simulink model "Final"  (R2018a)
settings: Solver=ode4  StartTime=0.0  StopTime=inf  FixedStep=0.01  RelTol=1e-3  EnableMultiTasking=on
model workspace (MAT data in the model file):
  Kp = 1
settings Model: ExtModeTrigDuration=5000  ParameterArgumentNames=Kp  OrderedModelArguments=off  Creator=benmiao  LastModifiedBy=benmiao
settings SolverCC: PositivePriorityOrder=on
settings DataIOCC: LimitDataPoints=on  SaveFormat=Array
settings OptimizationCC: ExpressionDepthLimit=2147483647  LifeSpan=inf
settings DebuggingCC: UnderspecifiedInitializationDetection=Classic  MergeDetectMultiDrivingBlocksExec=none  SolverPrmCheckMsg=warning  StateNameClashWarn=warning  SFUnexpectedBacktrackingDiag=warning  SFNoUnconditionalDefaultTransitionDiag=warning  SFExecutionAtInitializationDiag=none
settings HardwareCC: ProdBitPerPointer=32  ProdBitPerSizeT=32  ProdBitPerPtrDiffT=32  ProdLargestAtomicFloat=None  ProdIntDivRoundTo=Undefined  ProdEndianess=Unspecified  ProdWordSize=32  ProdHWDeviceType=32-bit Generic
settings ModelReferenceCC: PropagateSignalLabelsOutOfModel=off
settings RTWCC: SystemTargetFile=quarc_win64.tlc  TemplateMakefile=quarc_default_tmf  Description=QUARC Win64 Target
settings CodeAppCC: StateflowObjectComments=on
settings STFCustomTargetCC: TargetPreCompLibLocation=C:\PROGRA~3\QUARC\lib\2012b\win64\release  GeneratePreprocessorConditionals=Disable all  CombineOutputUpdateFcns=on  CPPClassGenCompliant=on  GRTInterface=off  SystemTargetFile=quarc_win64.tlc
settings GRTTargetCC: TargetPreCompLibLocation=C:\PROGRA~3\QUARC\lib\2012b\win64\release  TargetLangStandard=C89/C90 (ANSI)  ParMdlRefBuildCompliant=off  CompOptLevelCompliant=off  ConcurrentExecutionCompliant=off  GeneratePreprocessorConditionals=Disable all  MatFileLogging=off  UseToolchainInfoCompliant=off  ExtMode=on  ExtModeMexFile=quarc_comm
settings ConfigComp: CovMetricSettings=dw  CovHtmlReporting=on  CovSaveCumulativeToWorkspaceVar=on  CovSaveSingleToWorkspaceVar=on  CovExternalEMLEnable=off

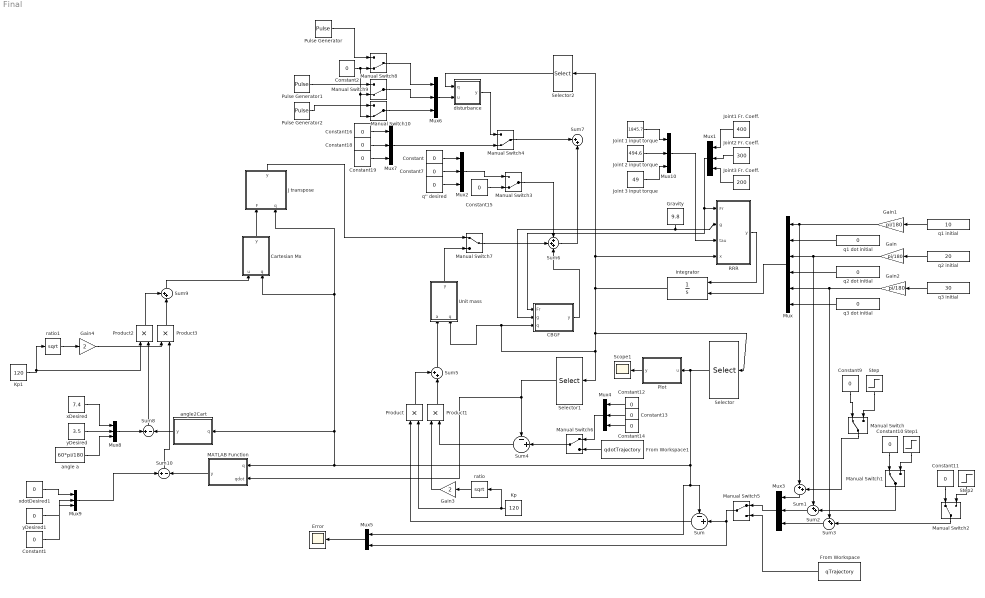
== system Final ==
  CBGF : MATLAB Function  TreatAsAtomicUnit=on
  Cartesian Mx : MATLAB Function  TreatAsAtomicUnit=on
  Constant{,1..2,7,9..16,18..19} (14 alike) : Constant  Value=0
  Error : Scope
  From Workspace : FromWorkspace  VariableName=qTrajectory  SampleTime=0
  From Workspace1 : FromWorkspace  VariableName=qdotTrajectory  SampleTime=0
  Gain : Gain  Gain=pi/180
  Gain1 : Gain  Gain=pi/180
  Gain2 : Gain  Gain=pi/180
  Gain3 : Gain  Gain=2
  Gain4 : Gain  Gain=2
  Gravity : Constant  Value=9.8
  Integrator : Integrator  InitialConditionSource=external
  J transpose : MATLAB Function  TreatAsAtomicUnit=on
  Joint 1 input torque : Constant  Value=1845.7
  Joint 2 input torque : Constant  Value=494.6
  Joint 3 input torque : Constant  Value=49
  Joint1 Fr. Coeff. : Constant  Value=400
  Joint2 Fr. Coeff. : Constant  Value=300
  Joint3 Fr. Coeff. : Constant  Value=200
  Kp : Constant  Value=120
  Kp1 : Constant  Value=120
  MATLAB Function : MATLAB Function  TreatAsAtomicUnit=on
  Manual Switch{,1..2,5..7} (6 alike) : ManualSwitch
  Manual Switch{3..4,8..10} (5 alike) : ManualSwitch  CurrentSetting=0
  Mux : Mux  Inputs=6
  Mux{1..4,6..10} (9 alike) : Mux  Inputs=3
  Mux5 : Mux  Inputs=2
  Plot : MATLAB Function  TreatAsAtomicUnit=on
  Product{,1..3} (4 alike) : Product
  Pulse Generator : DiscretePulseGenerator  PulseType=Time based  Amplitude=200  Period=5  PulseWidth=5
  Pulse Generator1 : DiscretePulseGenerator  PulseType=Time based  Amplitude=200  Period=5  PulseWidth=5
  Pulse Generator2 : DiscretePulseGenerator  PulseType=Time based  Amplitude=200  Period=5  PulseWidth=5
  RRR : MATLAB Function  TreatAsAtomicUnit=on
  Scope1 : Scope
  Selector : Selector  InputPortWidth=6  IndexOptions=Index vector (dialog)  Indices=[1 3 5]  OutputSizes=1
  Selector1 : Selector  InputPortWidth=6  IndexOptions=Index vector (dialog)  Indices=[2 4 6]  OutputSizes=1
  Selector2 : Selector  InputPortWidth=6  IndexOptions=Index vector (dialog)  Indices=[1 3 5]  OutputSizes=1
  Step : Step  Time=0  After=pi/18  SampleTime=0
  Step1 : Step  Time=0  After=pi/18  SampleTime=0
  Step2 : Step  Time=0  After=pi/2  SampleTime=0
  Sum : Sum  Inputs=-+|
  Sum1 : Sum  Inputs=|++
  Sum10 : Sum  Inputs=+|-
  Sum{2..3,5,9} (4 alike) : Sum  Inputs=++|
  Sum4 : Sum  Inputs=-+|
  Sum6 : Sum  Inputs=+++
  Sum7 : Sum  Inputs=|++
  Sum8 : Sum  Inputs=+|-
  Unit mass : MATLAB Function  TreatAsAtomicUnit=on
  angle a : Constant  Value=60*pi/180
  angle2Cart : MATLAB Function  TreatAsAtomicUnit=on
  disturbance : MATLAB Function  TreatAsAtomicUnit=on
  q'' desired : Constant  Value=0
  q1 dot initial : Constant  Value=0
  q1 initial : Constant  Value=10
  q2 dot initial : Constant  Value=0
  q2 initial : Constant  Value=20
  q3 dot initial : Constant  Value=0
  q3 initial : Constant  Value=30
  ratio : Sqrt  SaturateOnIntegerOverflow=on
  ratio1 : Sqrt  SaturateOnIntegerOverflow=on
  xDesired : Constant  Value=7.4
  xdotDesired1 : Constant  Value=0
  yDesired : Constant  Value=3.5
  yDesired1 : Constant  Value=0
  wires:
  q1 initial/1 -> Gain1/1
  q1 dot initial/1 -> Mux/2
  q2 dot initial/1 -> Mux/4
  q3 initial/1 -> Gain2/1
  q3 dot initial/1 -> Mux/6
  RRR/1(y) -> Integrator/1
  Gravity/1 -> CBGF/2(g), RRR/2(g)
  Selector/1 -> Sum/1, Mux5/1, Cartesian Mx/2(q), J transpose/2(q), angle2Cart/1(q), MATLAB Function/1(q), Plot/1(u)
  Integrator/1 -> Selector2/1, RRR/4(x), CBGF/3(q), Unit mass/2(q), Selector1/1, Selector/1
  Mux1/1 -> CBGF/1(Fr), RRR/1(Fr)
  Plot/1(y) -> Scope1/1
  Constant/1 -> Mux2/1
  Constant7/1 -> Mux2/2
  q'' desired/1 -> Mux2/3
  Mux/1 -> Integrator/2
  Joint1 Fr. Coeff./1 -> Mux1/1
  Joint2 Fr. Coeff./1 -> Mux1/2
  Joint3 Fr. Coeff./1 -> Mux1/3
  Sum/1 -> Product/1
  Step/1 -> Manual Switch/2
  Manual Switch/1 -> Sum1/2
  Constant9/1 -> Manual Switch/1
  Sum1/1 -> Mux3/1
  Constant10/1 -> Manual Switch1/1
  Step1/1 -> Manual Switch1/2
  Manual Switch1/1 -> Sum2/2
  Sum2/1 -> Mux3/2
  Constant11/1 -> Manual Switch2/1
  Step2/1 -> Manual Switch2/2
  Manual Switch2/1 -> Sum3/2
  Sum3/1 -> Mux3/3
  Constant12/1 -> Mux4/1
  Constant13/1 -> Mux4/2
  Constant14/1 -> Mux4/3
  Mux4/1 -> Manual Switch6/1
  Selector1/1 -> MATLAB Function/2(qdot), Sum4/1
  Gain1/1 -> Sum1/1, Mux/1
  q2 initial/1 -> Gain/1
  Gain/1 -> Mux/3, Sum2/1
  Gain2/1 -> Mux/5, Sum3/1
  Sum5/1 -> Unit mass/1(a)
  Unit mass/1(y) -> Manual Switch7/2
  CBGF/1(y) -> Sum6/3
  Mux2/1 -> Manual Switch3/1
  Sum4/1 -> Product1/2
  Kp/1 -> ratio/1, Product/2
  Product/1 -> Sum5/1
  Product1/1 -> Sum5/2
  Constant15/1 -> Manual Switch3/2
  Manual Switch3/1 -> Sum6/1
  Mux5/1 -> Error/1
  Gain3/1 -> Product1/1
  Sum6/1 -> Sum7/2
  Mux6/1 -> disturbance/2(u)
  Mux10/1 -> RRR/3(tau)
  ratio/1 -> Gain3/1
  Mux3/1 -> Manual Switch5/1
  Manual Switch5/1 -> Mux5/2, Sum/2
  From Workspace/1 -> Manual Switch5/2
  From Workspace1/1 -> Manual Switch6/2
  Manual Switch6/1 -> Sum4/2
  Selector2/1 -> disturbance/1(q)
  Mux7/1 -> Manual Switch4/2
  Constant18/1 -> Mux7/2
  Constant19/1 -> Mux7/3
  Constant16/1 -> Mux7/1
  disturbance/1(y) -> Manual Switch4/1
  Manual Switch4/1 -> Sum7/1
  Pulse Generator/1 -> Manual Switch8/1
  xDesired/1 -> Mux8/1
  yDesired/1 -> Mux8/2
  angle a/1 -> Mux8/3
  Mux8/1 -> Sum8/1
  angle2Cart/1(y) -> Sum8/2
  Cartesian Mx/1(y) -> J transpose/1(F)
  J transpose/1(y) -> Manual Switch7/1
  Manual Switch7/1 -> Sum6/2
  ratio1/1 -> Gain4/1
  Product3/1 -> Sum9/2
  Product2/1 -> Sum9/1
  Sum9/1 -> Cartesian Mx/1(u)
  Gain4/1 -> Product3/1
  MATLAB Function/1(y) -> Sum10/2
  xdotDesired1/1 -> Mux9/1
  Constant1/1 -> Mux9/3
  yDesired1/1 -> Mux9/2
  Mux9/1 -> Sum10/1
  Sum8/1 -> Product2/2
  Sum10/1 -> Product3/2
  Kp1/1 -> ratio1/1, Product2/1
  Pulse Generator1/1 -> Manual Switch9/1
  Pulse Generator2/1 -> Manual Switch10/1
  Manual Switch8/1 -> Mux6/1
  Manual Switch9/1 -> Mux6/2
  Manual Switch10/1 -> Mux6/3
  Constant2/1 -> Manual Switch9/2, Manual Switch10/2, Manual Switch8/2
  Joint 2 input torque/1 -> Mux10/2
  Joint 3 input torque/1 -> Mux10/3
  Joint 1 input torque/1 -> Mux10/1

== matlab function Final/Plot ==
  data: y output; u input
function y = fcn(u)
%
% q1 = u(1);
% q2 = u(2);
% q3 = u(3);
%
% x0 = 0;
% y0 = 0;
% x1 = 4*cos( q1);
% y1 = 4*sin( q1);
%
% x2 = 3*cos( (q1+q2));
% y2 = 3*sin( (q1+q2));
%
% x3 = 2*cos( (q1+q2+q3));
% y3 = 2*sin( (q1+q2+q3));
%
% px0= 0;
% py0 = 0;
% px1 = x1;
% py1 = y1;
% px2 = x1+x2;
% py2 = y1+y2;
% px3 = x1+x2+x3;
% py3 = y1+y2+y3;
%
% plot([px0,px1,px2,px3],[py0,py1,py2,py3]);
% xlim([-10,10]);
% ylim([-10,10]);
%
y = u;
q1 = u(1);
q2 = u(2);
q3 = u(3);
L1 = 4;
L2 = 3;
L3 = 2;

link11_end = [4;0;0;1];
link11_start = [0;0;0;1];
link22_end = [3;0;0;1];
link33_end = [2;0;0;1];
linkE3_end1 = [2;0.5;0;1];
linkE3_end2 = [2.5;0.5;0;1];
linkE3_end3 = [2;-0.5;0;1];
linkE3_end4 = [2.5;-0.5;0;1];


T_01 = [cos(q1) -sin(q1) 0 0;
    sin(q1) cos(q1) 0 0;
    0 0 1 0;
    0 0 0 1];

T_02 = [cos(q1+q2) -sin(q1+q2) 0 L1*cos(q1);
    sin(q1+q2) cos(q1+q2) 0 L1*sin(q1);
    0 0 1 0;
    0 0 0 1];

T_03 = [cos(q1+q2+q3) -sin(q1+q2+q3) 0 L2*cos(q1+q2)+L1*cos(q1);
    sin(q1+q2+q3) cos(q1+q2+q3) 0 L2*sin(q1+q2)+L1*sin(q1);
    0 0 1 0;
    0 0 0 1];

link10_end = T_01* link11_end;
link10_start = T_01* link11_start;

link20_end = T_02 * link22_end;

link30_end = T_03 * link33_end;

linkE0_end1 = T_03 * linkE3_end1;
linkE0_end2 = T_03 * linkE3_end2;
linkE0_end3 = T_03 * linkE3_end3;
linkE0_end4 = T_03 * linkE3_end4;

% plot([link10_start(1),link10_end(1),link20_end(1),link30_end(1),linkE0_end1(1),linkE0_end2(1),linkE0_end1(1),linkE0_end3(1),linkE0_end4(1)], ...
% [link10_start(2),link10_end(2),link20_end(2),link30_end(2),linkE0_end1(2),linkE0_end2(2),linkE0_end1(2),linkE0_end3(2),linkE0_end4(2)]);

plot([link10_start(1),link10_end(1)],[link10_start(2),link10_end(2)],'k');

hold on;
plot([link10_end(1),link20_end(1)],[link10_end(2),link20_end(2)],'m');

plot([link20_end(1),link30_end(1)],[link20_end(2),link30_end(2)],'b');

plot([link30_end(1),linkE0_end1(1),linkE0_end2(1),linkE0_end1(1),linkE0_end3(1),linkE0_end4(1)], ...
    [link30_end(2),linkE0_end1(2),linkE0_end2(2),linkE0_end1(2),linkE0_end3(2),linkE0_end4(2)],'c');

hold off;
grid on
xlim([-10,10]);
ylim([-10,10]);
title('RRR Robot Simulation');
xlabel('x Position');
ylabel('y Position');
end

== matlab function Final/RRR ==
  data: Fr input; g input; tau input; x input; y output

function y = fcn(Fr,g,tau,x)

q1 = x(1);
q2 = x(3);
q3 = x(5);

M = zeros(3);
M = [80*cos(q2 + q3) + 420*cos(q2) + 60*cos(q3) + 12291/20, 40*cos(q2 + q3) + 210*cos(q2) + 60*cos(q3) + 2681/20, 40*cos(q2 + q3) + 30*cos(q3) + 101/10;
    40*cos(q2 + q3) + 210*cos(q2) + 60*cos(q3) + 2681/20,                                 60*cos(q3) + 2681/20,                   30*cos(q3) + 101/10;
    40*cos(q2 + q3) + 30*cos(q3) + 101/10,                                  30*cos(q3) + 101/10,                                101/10];

B = zeros(3);
B = [ - 80*sin(q2 + q3) - 420*sin(q2), - 80*sin(q2 + q3) - 60*sin(q3), - 80*sin(q2 + q3) - 60*sin(q3);
    0,                    -60*sin(q3),                    -60*sin(q3);
    60*sin(q3),                              0,                              0];

C= zeros(3);
C = [                             0, - 40*sin(q2 + q3) - 210*sin(q2), - 40*sin(q2 + q3) - 30*sin(q3);
    40*sin(q2 + q3) + 210*sin(q2),                               0,                    -30*sin(q3);
    40*sin(q2 + q3) + 30*sin(q3),                      30*sin(q3),                              0];

G = [0;0;0];
G = [15*g*((3*cos(q1 + q2))/2 + 4*cos(q1)) + 10*g*(cos(q1 + q2 + q3) + 3*cos(q1 + q2) + 4*cos(q1)) + 40*g*cos(q1);
    10*g*(cos(q1 + q2 + q3) + 3*cos(q1 + q2)) + (45*g*cos(q1 + q2))/2;
    10*g*cos(q1 + q2 + q3)];

F = Fr .* [x(2);x(4);x(6)];

qdotdot = M\(tau -   C*[x(2)^2;x(4)^2;x(6)^2] - B*[ x(2)*x(4); x(2)*x(6); x(4)*x(6)] - G - F);
torque = C*[x(2)^2;x(4)^2;x(6)^2]+ B*[ x(2)*x(4); x(2)*x(6); x(4)*x(6)] + G

y = [x(2);
    qdotdot(1);
    x(4);
    qdotdot(2);
    x(6);
    qdotdot(3)];
end

== matlab function Final/Unit mass ==
  data: a input; y output; q input
function y = fcn(a,q)
q1 = q(1);
q2 = q(3);
q3 = q(5);

M = zeros(3);
M = [80*cos(q2 + q3) + 420*cos(q2) + 60*cos(q3) + 12291/20, 40*cos(q2 + q3) + 210*cos(q2) + 60*cos(q3) + 2681/20, 40*cos(q2 + q3) + 30*cos(q3) + 101/10;
    40*cos(q2 + q3) + 210*cos(q2) + 60*cos(q3) + 2681/20,                                 60*cos(q3) + 2681/20,                   30*cos(q3) + 101/10;
    40*cos(q2 + q3) + 30*cos(q3) + 101/10,                                  30*cos(q3) + 101/10,                                101/10];

y = M*a;
end

== matlab function Final/CBGF ==
  data: Fr input; y output; g input; q input
function y = fcn(Fr,g,q)
q1 = q(1);
q2 = q(3);
q3 = q(5);

M = zeros(3);
M = [80*cos(q2 + q3) + 420*cos(q2) + 60*cos(q3) + 12291/20, 40*cos(q2 + q3) + 210*cos(q2) + 60*cos(q3) + 2681/20, 40*cos(q2 + q3) + 30*cos(q3) + 101/10;
    40*cos(q2 + q3) + 210*cos(q2) + 60*cos(q3) + 2681/20,                                 60*cos(q3) + 2681/20,                   30*cos(q3) + 101/10;
    40*cos(q2 + q3) + 30*cos(q3) + 101/10,                                  30*cos(q3) + 101/10,                                101/10];

B = zeros(3);
B = [ - 80*sin(q2 + q3) - 420*sin(q2), - 80*sin(q2 + q3) - 60*sin(q3), - 80*sin(q2 + q3) - 60*sin(q3);
    0,                    -60*sin(q3),                    -60*sin(q3);
    60*sin(q3),                              0,                              0];

C= zeros(3);
C = [                             0, - 40*sin(q2 + q3) - 210*sin(q2), - 40*sin(q2 + q3) - 30*sin(q3);
    40*sin(q2 + q3) + 210*sin(q2),                               0,                    -30*sin(q3);
    40*sin(q2 + q3) + 30*sin(q3),                      30*sin(q3),                              0];

G = [0;0;0];
G = [15*g*((3*cos(q1 + q2))/2 + 4*cos(q1)) + 10*g*(cos(q1 + q2 + q3) + 3*cos(q1 + q2) + 4*cos(q1)) + 40*g*cos(q1);
    10*g*(cos(q1 + q2 + q3) + 3*cos(q1 + q2)) + (45*g*cos(q1 + q2))/2;
    10*g*cos(q1 + q2 + q3)];

F = Fr .* [q(2);q(4);q(6)];

y = C*[q(2)^2;q(4)^2;q(6)^2] + B*[ q(2)*q(4); q(2)*q(6); q(4)*q(6)] + G + F;

== matlab function Final/disturbance ==
  data: q input; u input; y output
function y = fcn(q,u)
L1 = 4;
L2 = 3;
L3 = 2;

q1 = q(1);
q2 = q(2);
q3 = q(3);

J0 = [-L3*sin(q1+q2+q3)-L2*sin(q1+q2)-L1*sin(q1) -L3*sin(q1+q2+q3)-L2*sin(q1+q2) -L3*sin(q1+q2+q3);
    L3*cos(q1+q2+q3)+L2*cos(q1+q2)+L1*cos(q1) L3*cos(q1+q2+q3)+L2*cos(q1+q2) L3*cos(q1+q2+q3);
    1 0 0];


y = J0.' * u;

== matlab function Final/Cartesian Mx ==
  data: u input; y output; q input
function y = mx(u,q)
q1 = q(1);
q2 = q(2);
q3 = q(3);
Mx = [                                                                                                                                                                                                                                                                                                                                                                                                                                                                                (((101*(2*cos(q1 + q2 + q3) + 3*cos(q1 + q2)))/(60*(cos(q1 + q2 + q3)*sin(q1 + q2) - sin(q1 + q2 + q3)*cos(q1 + q2))) - (cos(q1 + q2 + q3)*(30*cos(q3) + 101/10))/(3*(cos(q1 + q2 + q3)*sin(q1 + q2) - sin(q1 + q2 + q3)*cos(q1 + q2))))*(2*cos(q1 + q2 + q3) + 3*cos(q1 + q2)))/(6*(cos(q1 + q2 + q3)*sin(q1 + q2) - sin(q1 + q2 + q3)*cos(q1 + q2))) + (cos(q1 + q2 + q3)*((cos(q1 + q2 + q3)*(60*cos(q3) + 2681/20))/(3*(cos(q1 + q2 + q3)*sin(q1 + q2) - sin(q1 + q2 + q3)*cos(q1 + q2))) - ((30*cos(q3) + 101/10)*(2*cos(q1 + q2 + q3) + 3*cos(q1 + q2)))/(6*(cos(q1 + q2 + q3)*sin(q1 + q2) - sin(q1 + q2 + q3)*cos(q1 + q2)))))/(3*(cos(q1 + q2 + q3)*sin(q1 + q2) - sin(q1 + q2 + q3)*cos(q1 + q2))),                                                                                                                                                                                                                                                                                                                                                                                                                                                                                (((101*(2*cos(q1 + q2 + q3) + 3*cos(q1 + q2)))/(60*(cos(q1 + q2 + q3)*sin(q1 + q2) - sin(q1 + q2 + q3)*cos(q1 + q2))) - (cos(q1 + q2 + q3)*(30*cos(q3) + 101/10))/(3*(cos(q1 + q2 + q3)*sin(q1 + q2) - sin(q1 + q2 + q3)*cos(q1 + q2))))*(2*sin(q1 + q2 + q3) + 3*sin(q1 + q2)))/(6*(cos(q1 + q2 + q3)*sin(q1 + q2) - sin(q1 + q2 + q3)*cos(q1 + q2))) + (sin(q1 + q2 + q3)*((cos(q1 + q2 + q3)*(60*cos(q3) + 2681/20))/(3*(cos(q1 + q2 + q3)*sin(q1 + q2) - sin(q1 + q2 + q3)*cos(q1 + q2))) - ((30*cos(q3) + 101/10)*(2*cos(q1 + q2 + q3) + 3*cos(q1 + q2)))/(6*(cos(q1 + q2 + q3)*sin(q1 + q2) - sin(q1 + q2 + q3)*cos(q1 + q2)))))/(3*(cos(q1 + q2 + q3)*sin(q1 + q2) - sin(q1 + q2 + q3)*cos(q1 + q2))),                                                                                                                                                                                                                                                                                                                                                                                                                                                                                                                                                                                                                                                                                                                                 (2*((101*(2*cos(q1 + q2 + q3) + 3*cos(q1 + q2)))/(60*(cos(q1 + q2 + q3)*sin(q1 + q2) - sin(q1 + q2 + q3)*cos(q1 + q2))) - (cos(q1 + q2 + q3)*(30*cos(q3) + 101/10))/(3*(cos(q1 + q2 + q3)*sin(q1 + q2) - sin(q1 + q2 + q3)*cos(q1 + q2))))*(2*cos(q1 + q2 + q3)*sin(q1) - 2*sin(q1 + q2 + q3)*cos(q1) + 3*cos(q1 + q2)*sin(q1) - 3*sin(q1 + q2)*cos(q1)))/(3*(cos(q1 + q2 + q3)*sin(q1 + q2) - sin(q1 + q2 + q3)*cos(q1 + q2))) + (((cos(q1 + q2 + q3)*(60*cos(q3) + 2681/20))/(3*(cos(q1 + q2 + q3)*sin(q1 + q2) - sin(q1 + q2 + q3)*cos(q1 + q2))) - ((30*cos(q3) + 101/10)*(2*cos(q1 + q2 + q3) + 3*cos(q1 + q2)))/(6*(cos(q1 + q2 + q3)*sin(q1 + q2) - sin(q1 + q2 + q3)*cos(q1 + q2))))*(3*cos(q1 + q2 + q3)*sin(q1 + q2) - 3*sin(q1 + q2 + q3)*cos(q1 + q2) + 4*cos(q1 + q2 + q3)*sin(q1) - 4*sin(q1 + q2 + q3)*cos(q1)))/(3*(cos(q1 + q2 + q3)*sin(q1 + q2) - sin(q1 + q2 + q3)*cos(q1 + q2))) - (cos(q1 + q2 + q3)*(40*cos(q2 + q3) + 210*cos(q2) + 60*cos(q3) + 2681/20))/(3*(cos(q1 + q2 + q3)*sin(q1 + q2) - sin(q1 + q2 + q3)*cos(q1 + q2))) + ((2*cos(q1 + q2 + q3) + 3*cos(q1 + q2))*(40*cos(q2 + q3) + 30*cos(q3) + 101/10))/(6*(cos(q1 + q2 + q3)*sin(q1 + q2) - sin(q1 + q2 + q3)*cos(q1 + q2)));
                                                                                                                                                                                                                                                                                                                                                                                                                                                                                (cos(q1 + q2 + q3)*((sin(q1 + q2 + q3)*(60*cos(q3) + 2681/20))/(3*(cos(q1 + q2 + q3)*sin(q1 + q2) - sin(q1 + q2 + q3)*cos(q1 + q2))) - ((30*cos(q3) + 101/10)*(2*sin(q1 + q2 + q3) + 3*sin(q1 + q2)))/(6*(cos(q1 + q2 + q3)*sin(q1 + q2) - sin(q1 + q2 + q3)*cos(q1 + q2)))))/(3*(cos(q1 + q2 + q3)*sin(q1 + q2) - sin(q1 + q2 + q3)*cos(q1 + q2))) + ((2*cos(q1 + q2 + q3) + 3*cos(q1 + q2))*((101*(2*sin(q1 + q2 + q3) + 3*sin(q1 + q2)))/(60*(cos(q1 + q2 + q3)*sin(q1 + q2) - sin(q1 + q2 + q3)*cos(q1 + q2))) - (sin(q1 + q2 + q3)*(30*cos(q3) + 101/10))/(3*(cos(q1 + q2 + q3)*sin(q1 + q2) - sin(q1 + q2 + q3)*cos(q1 + q2)))))/(6*(cos(q1 + q2 + q3)*sin(q1 + q2) - sin(q1 + q2 + q3)*cos(q1 + q2))),                                                                                                                                                                                                                                                                                                                                                                                                                                                                                (sin(q1 + q2 + q3)*((sin(q1 + q2 + q3)*(60*cos(q3) + 2681/20))/(3*(cos(q1 + q2 + q3)*sin(q1 + q2) - sin(q1 + q2 + q3)*cos(q1 + q2))) - ((30*cos(q3) + 101/10)*(2*sin(q1 + q2 + q3) + 3*sin(q1 + q2)))/(6*(cos(q1 + q2 + q3)*sin(q1 + q2) - sin(q1 + q2 + q3)*cos(q1 + q2)))))/(3*(cos(q1 + q2 + q3)*sin(q1 + q2) - sin(q1 + q2 + q3)*cos(q1 + q2))) + (((101*(2*sin(q1 + q2 + q3) + 3*sin(q1 + q2)))/(60*(cos(q1 + q2 + q3)*sin(q1 + q2) - sin(q1 + q2 + q3)*cos(q1 + q2))) - (sin(q1 + q2 + q3)*(30*cos(q3) + 101/10))/(3*(cos(q1 + q2 + q3)*sin(q1 + q2) - sin(q1 + q2 + q3)*cos(q1 + q2))))*(2*sin(q1 + q2 + q3) + 3*sin(q1 + q2)))/(6*(cos(q1 + q2 + q3)*sin(q1 + q2) - sin(q1 + q2 + q3)*cos(q1 + q2))),                                                                                                                                                                                                                                                                                                                                                                                                                                                                                                                                                                                                                                                                                                                                 ((2*sin(q1 + q2 + q3) + 3*sin(q1 + q2))*(40*cos(q2 + q3) + 30*cos(q3) + 101/10))/(6*(cos(q1 + q2 + q3)*sin(q1 + q2) - sin(q1 + q2 + q3)*cos(q1 + q2))) + (2*((101*(2*sin(q1 + q2 + q3) + 3*sin(q1 + q2)))/(60*(cos(q1 + q2 + q3)*sin(q1 + q2) - sin(q1 + q2 + q3)*cos(q1 + q2))) - (sin(q1 + q2 + q3)*(30*cos(q3) + 101/10))/(3*(cos(q1 + q2 + q3)*sin(q1 + q2) - sin(q1 + q2 + q3)*cos(q1 + q2))))*(2*cos(q1 + q2 + q3)*sin(q1) - 2*sin(q1 + q2 + q3)*cos(q1) + 3*cos(q1 + q2)*sin(q1) - 3*sin(q1 + q2)*cos(q1)))/(3*(cos(q1 + q2 + q3)*sin(q1 + q2) - sin(q1 + q2 + q3)*cos(q1 + q2))) + (((sin(q1 + q2 + q3)*(60*cos(q3) + 2681/20))/(3*(cos(q1 + q2 + q3)*sin(q1 + q2) - sin(q1 + q2 + q3)*cos(q1 + q2))) - ((30*cos(q3) + 101/10)*(2*sin(q1 + q2 + q3) + 3*sin(q1 + q2)))/(6*(cos(q1 + q2 + q3)*sin(q1 + q2) - sin(q1 + q2 + q3)*cos(q1 + q2))))*(3*cos(q1 + q2 + q3)*sin(q1 + q2) - 3*sin(q1 + q2 + q3)*cos(q1 + q2) + 4*cos(q1 + q2 + q3)*sin(q1) - 4*sin(q1 + q2 + q3)*cos(q1)))/(3*(cos(q1 + q2 + q3)*sin(q1 + q2) - sin(q1 + q2 + q3)*cos(q1 + q2))) - (sin(q1 + q2 + q3)*(40*cos(q2 + q3) + 210*cos(q2) + 60*cos(q3) + 2681/20))/(3*(cos(q1 + q2 + q3)*sin(q1 + q2) - sin(q1 + q2 + q3)*cos(q1 + q2)));
 ((2*cos(q1 + q2 + q3) + 3*cos(q1 + q2))*(40*cos(q2 + q3) + 30*cos(q3) + (101*(2*cos(q1 + q2 + q3)*sin(q1) - 2*sin(q1 + q2 + q3)*cos(q1) + 3*cos(q1 + q2)*sin(q1) - 3*sin(q1 + q2)*cos(q1)))/(15*(cos(q1 + q2 + q3)*sin(q1 + q2) - sin(q1 + q2 + q3)*cos(q1 + q2))) - ((30*cos(q3) + 101/10)*(3*cos(q1 + q2 + q3)*sin(q1 + q2) - 3*sin(q1 + q2 + q3)*cos(q1 + q2) + 4*cos(q1 + q2 + q3)*sin(q1) - 4*sin(q1 + q2 + q3)*cos(q1)))/(3*(cos(q1 + q2 + q3)*sin(q1 + q2) - sin(q1 + q2 + q3)*cos(q1 + q2))) + 101/10))/(6*(cos(q1 + q2 + q3)*sin(q1 + q2) - sin(q1 + q2 + q3)*cos(q1 + q2))) - (cos(q1 + q2 + q3)*(40*cos(q2 + q3) + 210*cos(q2) + 60*cos(q3) - ((60*cos(q3) + 2681/20)*(3*cos(q1 + q2 + q3)*sin(q1 + q2) - 3*sin(q1 + q2 + q3)*cos(q1 + q2) + 4*cos(q1 + q2 + q3)*sin(q1) - 4*sin(q1 + q2 + q3)*cos(q1)))/(3*(cos(q1 + q2 + q3)*sin(q1 + q2) - sin(q1 + q2 + q3)*cos(q1 + q2))) + (2*(30*cos(q3) + 101/10)*(2*cos(q1 + q2 + q3)*sin(q1) - 2*sin(q1 + q2 + q3)*cos(q1) + 3*cos(q1 + q2)*sin(q1) - 3*sin(q1 + q2)*cos(q1)))/(3*(cos(q1 + q2 + q3)*sin(q1 + q2) - sin(q1 + q2 + q3)*cos(q1 + q2))) + 2681/20))/(3*(cos(q1 + q2 + q3)*sin(q1 + q2) - sin(q1 + q2 + q3)*cos(q1 + q2))), ((2*sin(q1 + q2 + q3) + 3*sin(q1 + q2))*(40*cos(q2 + q3) + 30*cos(q3) + (101*(2*cos(q1 + q2 + q3)*sin(q1) - 2*sin(q1 + q2 + q3)*cos(q1) + 3*cos(q1 + q2)*sin(q1) - 3*sin(q1 + q2)*cos(q1)))/(15*(cos(q1 + q2 + q3)*sin(q1 + q2) - sin(q1 + q2 + q3)*cos(q1 + q2))) - ((30*cos(q3) + 101/10)*(3*cos(q1 + q2 + q3)*sin(q1 + q2) - 3*sin(q1 + q2 + q3)*cos(q1 + q2) + 4*cos(q1 + q2 + q3)*sin(q1) - 4*sin(q1 + q2 + q3)*cos(q1)))/(3*(cos(q1 + q2 + q3)*sin(q1 + q2) - sin(q1 + q2 + q3)*cos(q1 + q2))) + 101/10))/(6*(cos(q1 + q2 + q3)*sin(q1 + q2) - sin(q1 + q2 + q3)*cos(q1 + q2))) - (sin(q1 + q2 + q3)*(40*cos(q2 + q3) + 210*cos(q2) + 60*cos(q3) - ((60*cos(q3) + 2681/20)*(3*cos(q1 + q2 + q3)*sin(q1 + q2) - 3*sin(q1 + q2 + q3)*cos(q1 + q2) + 4*cos(q1 + q2 + q3)*sin(q1) - 4*sin(q1 + q2 + q3)*cos(q1)))/(3*(cos(q1 + q2 + q3)*sin(q1 + q2) - sin(q1 + q2 + q3)*cos(q1 + q2))) + (2*(30*cos(q3) + 101/10)*(2*cos(q1 + q2 + q3)*sin(q1) - 2*sin(q1 + q2 + q3)*cos(q1) + 3*cos(q1 + q2)*sin(q1) - 3*sin(q1 + q2)*cos(q1)))/(3*(cos(q1 + q2 + q3)*sin(q1 + q2) - sin(q1 + q2 + q3)*cos(q1 + q2))) + 2681/20))/(3*(cos(q1 + q2 + q3)*sin(q1 + q2) - sin(q1 + q2 + q3)*cos(q1 + q2))), 80*cos(q2 + q3) + 420*cos(q2) + 60*cos(q3) - ((3*cos(q1 + q2 + q3)*sin(q1 + q2) - 3*sin(q1 + q2 + q3)*cos(q1 + q2) + 4*cos(q1 + q2 + q3)*sin(q1) - 4*sin(q1 + q2 + q3)*cos(q1))*(40*cos(q2 + q3) + 210*cos(q2) + 60*cos(q3) + 2681/20))/(3*(cos(q1 + q2 + q3)*sin(q1 + q2) - sin(q1 + q2 + q3)*cos(q1 + q2))) + (2*(2*cos(q1 + q2 + q3)*sin(q1) - 2*sin(q1 + q2 + q3)*cos(q1) + 3*cos(q1 + q2)*sin(q1) - 3*sin(q1 + q2)*cos(q1))*(40*cos(q2 + q3) + 30*cos(q3) + (101*(2*cos(q1 + q2 + q3)*sin(q1) - 2*sin(q1 + q2 + q3)*cos(q1) + 3*cos(q1 + q2)*sin(q1) - 3*sin(q1 + q2)*cos(q1)))/(15*(cos(q1 + q2 + q3)*sin(q1 + q2) - sin(q1 + q2 + q3)*cos(q1 + q2))) - ((30*cos(q3) + 101/10)*(3*cos(q1 + q2 + q3)*sin(q1 + q2) - 3*sin(q1 + q2 + q3)*cos(q1 + q2) + 4*cos(q1 + q2 + q3)*sin(q1) - 4*sin(q1 + q2 + q3)*cos(q1)))/(3*(cos(q1 + q2 + q3)*sin(q1 + q2) - sin(q1 + q2 + q3)*cos(q1 + q2))) + 101/10))/(3*(cos(q1 + q2 + q3)*sin(q1 + q2) - sin(q1 + q2 + q3)*cos(q1 + q2))) + (2*(40*cos(q2 + q3) + 30*cos(q3) + 101/10)*(2*cos(q1 + q2 + q3)*sin(q1) - 2*sin(q1 + q2 + q3)*cos(q1) + 3*cos(q1 + q2)*sin(q1) - 3*sin(q1 + q2)*cos(q1)))/(3*(cos(q1 + q2 + q3)*sin(q1 + q2) - sin(q1 + q2 + q3)*cos(q1 + q2))) - ((3*cos(q1 + q2 + q3)*sin(q1 + q2) - 3*sin(q1 + q2 + q3)*cos(q1 + q2) + 4*cos(q1 + q2 + q3)*sin(q1) - 4*sin(q1 + q2 + q3)*cos(q1))*(40*cos(q2 + q3) + 210*cos(q2) + 60*cos(q3) - ((60*cos(q3) + 2681/20)*(3*cos(q1 + q2 + q3)*sin(q1 + q2) - 3*sin(q1 + q2 + q3)*cos(q1 + q2) + 4*cos(q1 + q2 + q3)*sin(q1) - 4*sin(q1 + q2 + q3)*cos(q1)))/(3*(cos(q1 + q2 + q3)*sin(q1 + q2) - sin(q1 + q2 + q3)*cos(q1 + q2))) + (2*(30*cos(q3) + 101/10)*(2*cos(q1 + q2 + q3)*sin(q1) - 2*sin(q1 + q2 + q3)*cos(q1) + 3*cos(q1 + q2)*sin(q1) - 3*sin(q1 + q2)*cos(q1)))/(3*(cos(q1 + q2 + q3)*sin(q1 + q2) - sin(q1 + q2 + q3)*cos(q1 + q2))) + 2681/20))/(3*(cos(q1 + q2 + q3)*sin(q1 + q2) - sin(q1 + q2 + q3)*cos(q1 + q2))) + 12291/20];
y = Mx * u;

end

== matlab function Final/angle2Cart ==
  data: q input; y output
function y =  ang2Cart(q)
q1 = q(1);
q2 = q(2);
q3 = q(3);

L1 = 4;
L2 = 3;
L3 = 2;

T_0E = [cos(q1+q2+q3) -sin(q1+q2+q3) 0 L3*cos(q1+q2+q3)+L2*cos(q1+q2)+L1*cos(q1);
    sin(q1+q2+q3) cos(q1+q2+q3) 0 L3*sin(q1+q2+q3)+L2*sin(q1+q2)+L1*sin(q1);
    0 0 1 0;
    0 0 0 1];

Xpos= T_0E(1,4);
Ypos= T_0E(2,4);
a = atan2(T_0E(2,1),T_0E(1,1));
% a = atan(T_0E(2,1)/T_0E(1,1));
y = [Xpos, Ypos,a];

== matlab function Final/J transpose ==
  data: F input; q input; y output
function y = force2torque(F,q)
L1 = 4;
L2 = 3;
L3 = 2;

q1 = q(1);
q2 = q(2);
q3 = q(3);

J0 = [-L3*sin(q1+q2+q3)-L2*sin(q1+q2)-L1*sin(q1) -L3*sin(q1+q2+q3)-L2*sin(q1+q2) -L3*sin(q1+q2+q3);
    L3*cos(q1+q2+q3)+L2*cos(q1+q2)+L1*cos(q1) L3*cos(q1+q2+q3)+L2*cos(q1+q2) L3*cos(q1+q2+q3);
    1 0 0];


y = J0.' * F;

== matlab function Final/MATLAB Function ==
  data: q input; qdot input; y output
function y = xdot(q,qdot)
L1 = 4;
L2 = 3;
L3 = 2;

q1 = q(1);
q2 = q(2);
q3 = q(3);

J0 = [-L3*sin(q1+q2+q3)-L2*sin(q1+q2)-L1*sin(q1) -L3*sin(q1+q2+q3)-L2*sin(q1+q2) -L3*sin(q1+q2+q3);
    L3*cos(q1+q2+q3)+L2*cos(q1+q2)+L1*cos(q1) L3*cos(q1+q2+q3)+L2*cos(q1+q2) L3*cos(q1+q2+q3);
    1 0 0];

y = J0*qdot;
